simulink model "Torso"  (R2020b)
settings: Solver=FixedStepAuto  StartTime=0.0  StopTime=90  RelTol=1e-3
undefined symbols (not defined in the file): DiscIntNeverNeededParam
libraries: dspfdesign x2, androidsensorlib x1, vrlib x1
settings Model: SimulationMode=external  Creator=sarar  LastModifiedBy=sarar
settings DataIOCC: LimitDataPoints=on  SaveFinalState=on  SaveState=on  LoggingFileName=TorsoData.mat
settings OptimizationCC: EnhancedBackFolding=on  PassReuseOutputArgsAs=Individual arguments  ZeroExternalMemoryAtStartup=off  ZeroInternalMemoryAtStartup=off  MaxStackSize=64  OptimizeBlockOrder=speed  DifferentSizesBufferReuse=on  OptimizationCustomize=off  EfficientTunableParamExpr=on
settings DebuggingCC: ParameterTunabilityLossMsg=error
settings HardwareCC: ProdBitPerPointer=32  ProdBitPerSizeT=32  ProdBitPerPtrDiffT=32  ProdLargestAtomicInteger=Long  ProdLargestAtomicFloat=Double  ProdWordSize=32  ProdHWDeviceType=ARM Compatible->ARM Cortex
settings SFSimCC: MATLABDynamicMemAlloc=off
settings RTWCC: Description=Embedded Coder  SystemTargetFile=ert.tlc  HardwareBoard=Android Device  TLCOptions="-aInlineSetEventsForThisBaseRateFcn=TLC_FALSE -aSuppressMultiTaskScheduler=TLC_FALSE  -aRateBasedStepFcn=0"  TemplateMakefile=ert_default_tmf  RTWVerbose=off  Toolchain=Android SDK/NDK Tools
settings CodeAppCC: ForceParamTrailComments=on  IgnoreCustomStorageClasses=off  OperatorAnnotations=on  SimulinkDataObjDesc=on  SFDataObjDesc=on  InsertBlockDesc=on
settings ERTTargetCC: MatFileLogging=on

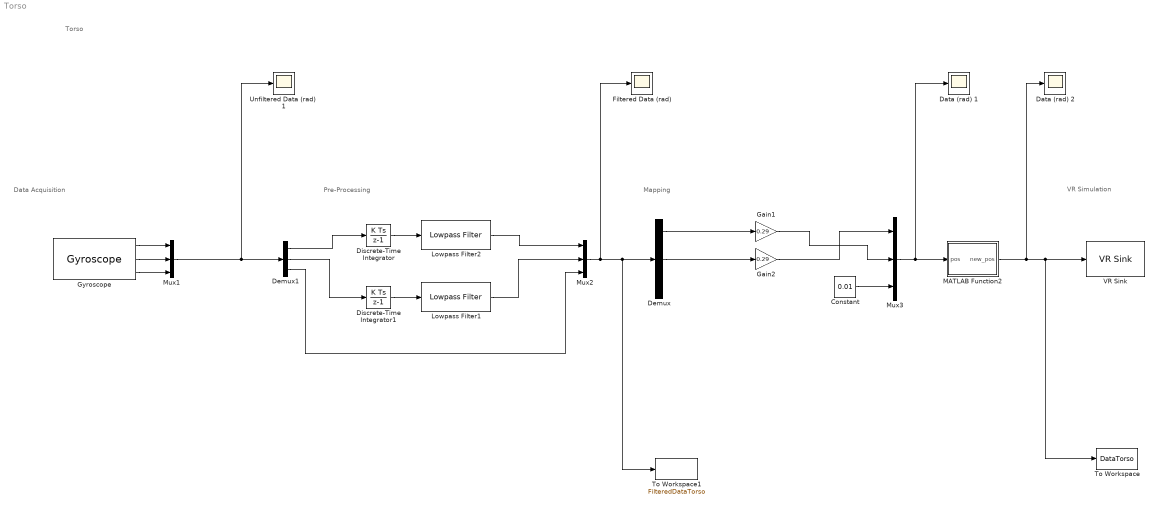
== system Torso ==
  note: Pre-Processing
  note: Torso
  note: VR Simulation
  note: Mapping
  note: Data Acquisition
  Constant : Constant  Value=0.01
  Data (rad) 1 : Scope
  Data (rad) 2 : Scope
  Demux : Demux  Outputs=3
  Demux1 : Demux  Outputs=3
  Discrete-Time Integrator : DiscreteIntegrator  SampleTime=-1  ICPrevOutput=DiscIntNeverNeededParam  ICPrevScaledInput=DiscIntNeverNeededParam
  Discrete-Time Integrator1 : DiscreteIntegrator  SampleTime=-1  ICPrevOutput=DiscIntNeverNeededParam  ICPrevScaledInput=DiscIntNeverNeededParam
  "Filtered Data (rad)  " : Scope
  Gain1 : Gain  Gain=0.29  OutDataTypeStr=Inherit: Inherit via back propagation
  Gain2 : Gain  Gain=0.29  OutDataTypeStr=Inherit: Inherit via back propagation
  Gyroscope : androidsensorlib/Gyroscope  OutputVector=off  SampleTime=0.016  BlockPlatform=Android
      settings: SourceProductBaseCode=ANDROID
  Lowpass Filter1 : dspfdesign/Lowpass Filter  FilterType=FIR  DesignForMinimumOrder=on  FilterOrder=5  PassbandFrequency=7  StopbandFrequency=10  PassbandRipple=0.1  StopbandAttenuation=50  InheritSampleRate=off  SampleRate=60  SimulateUsing=Interpreted execution  roundingMode=Floor  coeffsDataTypeStr=fixdt(1,16)
  Lowpass Filter2 : dspfdesign/Lowpass Filter  FilterType=FIR  DesignForMinimumOrder=on  FilterOrder=5  PassbandFrequency=7  StopbandFrequency=10  PassbandRipple=0.1  StopbandAttenuation=50  InheritSampleRate=off  SampleRate=60  SimulateUsing=Interpreted execution  roundingMode=Floor  coeffsDataTypeStr=fixdt(1,16)
  MATLAB Function2 : MATLAB Function  TreatAsAtomicUnit=on
  Mux1 : Mux  Inputs=3
  Mux2 : Mux  Inputs=3
  Mux3 : Mux  Inputs=3
  To Workspace : ToWorkspace  VariableName=DataTorso  SaveFormat=Structure  SampleTime=-1
  To Workspace1 : ToWorkspace  VariableName=FilteredDataTorso  SaveFormat=Structure  SampleTime=-1
  Unfiltered Data (rad)  1 : Scope
  VR Sink : vrlib/VR Sink  InstantiateOnLoad=on  SampleTime=0.1  ViewEnable=on  RemoteChange=off  RemoteView=off  FieldsWritten=cursor.translation.3.1.1.double  WorldFileName=8_palline_color.wrl  AutoView=on  VideoDimensions=[]  AllowVariableSize=off
  wires:
  Demux/1 -> Gain1/1
  Demux/2 -> Gain2/1
  Constant/1 -> Mux3/3
  Gain2/1 -> Mux3/1
  Gain1/1 -> Mux3/2
  Mux3/1 -> Data (rad) 1/1, MATLAB Function2/1(pos)
  MATLAB Function2/1(new_pos) -> To Workspace/1, VR Sink/1, Data (rad) 2/1
  Lowpass Filter2/1 -> Mux2/1
  Mux2/1 -> To Workspace1/1, Demux/1, "Filtered Data (rad)  "/1
  Gyroscope/2 -> Mux1/2
  Gyroscope/1 -> Mux1/1
  Gyroscope/3 -> Mux1/3
  Mux1/1 -> Demux1/1, Unfiltered Data (rad)  1/1
  Demux1/1 -> Discrete-Time Integrator/1
  Demux1/2 -> Discrete-Time Integrator1/1
  Demux1/3 -> Mux2/3
  Lowpass Filter1/1 -> Mux2/2
  Discrete-Time Integrator/1 -> Lowpass Filter2/1
  Discrete-Time Integrator1/1 -> Lowpass Filter1/1

== matlab function Torso/MATLAB Function2 ==
  data: pos input; new_pos output
function new_pos = map(pos)

new_pos = double(pos); 
%define theta 
theta = atan2(pos(2),pos(1)); 


if norm(pos(1)) > norm(0.1*cos(theta))
    new_pos(1) = 0.1 * cos(theta)   
else
    new_pos(1) = pos(1)
end

if norm(pos(2)) > norm(0.1*sin(theta))
    new_pos(2) = 0.1 * sin(theta) 
else
    new_pos(2) = pos(2) 
end 

new_pos(3) = pos(3) 


end
